simulink library "tqd"  (R2021b)
settings: Solver=VariableStepAuto  StartTime=0.0  StopTime=10.0  RelTol=1e-3
undefined symbols (not defined in the file): ATQD_AfterTqMinGain_X_Deg, ATQD_APSCreepBaseTqD_X_kph, ATQD_APSCreepBaseTqD_Y_Deg, ATQD_APSCreepBaseTqR_X_kph, ATQD_APSCreepBaseTqR_Y_Deg, ATQD_APSCreepIterm_X_kph, ATQD_APSCreepIterm_Y_kph, ATQD_APSCreepPterm_X_kph, ATQD_APSCreepPterm_Y_kph, ATQD_APSDecReq_X_kph, ATQD_APSDecReq_Y_mps2, ATQD_APSDecReqCMD_X_kph, ATQD_APSDecReqTs_X_pct, ATQD_APSDecTimeGain_X_Deg, ATQD_APSDecTimeGain_Y_s, ATQD_APSReqLowSpd_X_Deg, ATQD_AutoHoldReleaseBPS_X_Deg, ATQD_AWDLoadTrqnsGain_X_kg, ATQD_AWDLoadTrqnsGain_Y_pct, ATQD_BOSEnBPSPosn_X_kph, ATQD_BOSMap_X_rpm, ATQD_BOSMap_Y_pct, ATQD_CreepBaseTqD_X_kph, ATQD_CreepBaseTqD_Y_Deg, ATQD_CreepBaseTqR_X_kph, ATQD_CreepBaseTqR_Y_Deg, ATQD_CreepBPSDisPosn_X_Deg, ATQD_CreepBPSDisPosnR_X_Deg, ATQD_CreepBPSEnPosn_X_Deg, ATQD_CreepBPSEnPosnR_X_Deg, ATQD_CreepDeltaTq_X_kph, ATQD_CreepIterm_X_kph, ATQD_CreepIterm_Y_kph, ATQD_CreepItermMaxLimit_X_pct, ATQD_CreepPreloadTime_X_kph, ATQD_CreepPreloadTq_X_kph, ATQD_CreepPreloadTq_Y_s, ATQD_CreepProtTq_X_Deg, ATQD_CreepPterm_X_kph, ATQD_CreepPterm_Y_kph, ATQD_CreepRrTqSpRat_X_rpm, ATQD_CreepRrTqSpRat_Y_Nm, ATQD_CreepTargetSpdD_X_pct, ATQD_CreepTargetSpdR_X_pct, ATQD_ECOTqMapD_X_rpm, ATQD_ECOTqMapD_Y_pct, ATQD_EMTqMapD_X_rpm, ATQD_EMTqMapD_Y_pct, ATQD_EOPDTqMapDCon_X_rpm, ATQD_EOPDTqMapDCon_Y_Deg, ATQD_EscapeModePedTq_X_pct, ATQD_EscapeModePedTq_Y_rpm, ATQD_EscapeModePedTqFr_X_pct, ATQD_EscapeModePedTqFr_Y_rpm, ATQD_EstInitVehWeight_X_c, ATQD_FAfterTqCMDGain_X_rpm, ATQD_FAfterTqCMDGain_Y_pct, ATQD_FrLossMAPLowV_X_rpm, ATQD_FrLossMAPLowV_Y_Nm, ATQD_FrMotActReduce_X_rpm ... (+772)
libraries: simulink x211, hcu_lib x179, tqr x3
(part 26 of 28)

== stateflow chart tqd/TQD/TorqueDemand/Signal_convert/Chart ==
  state Creep_function_switch
    (default) -> (junction 12) : { VTQD_SaveCreepSW_flg =FALSE;}
    Creep_function_switch -> (junction 12)
    (junction 12) -> (junction 16) [order 1] : [VPMM_SysPowerMode_enum != ENUM_PWRSTASW_STANDBY ]
    (junction 12) -> (junction 19) [order 2] : {VTQD_CreepON_flg = TRUE;
        |  VTQD_SaveCreepSW_flg = VTQD_CreepON_flg;}
    (junction 16) -> (junction 23)
    (junction 23) -> (junction 25) [order 1] : [KTQD_CreepSW_flg_ovrdflg != TRUE]
    (junction 23) -> (junction 28) [order 2] : {VTQD_CreepON_flg = KTQD_CreepSW_flg_ovrdval;}
    (junction 25) -> (junction 30)
    (junction 30) -> (junction 32) [order 1] : [VINP_RegenMode_enum != ENUM_REGENLEVEL_OPD]
    (junction 30) -> (junction 34) [order 2] : {VTQD_CreepON_flg = FALSE;}
    (junction 32) -> (junction 37)
    (junction 37) -> (junction 39) [order 1] : [VTQD_OPDOn2Off_flg != TRUE]
    (junction 37) -> (junction 42) [order 2] : {VTQD_CreepON_flg = VTQD_SaveCreepSW_flg;}
    (junction 39) -> (junction 45)
    (junction 45) -> (junction 47) [order 1] : [VINP_IVICreepSWReq_flg == TRUE]
    (junction 45) -> (junction 49) [order 2] : {VTQD_CreepON_flg = VTQD_LastCreepON_flg;}
    (junction 47) -> (junction 51)
    (junction 51) -> (junction 53) [order 1] : [VTQD_LastCreepON_flg != FALSE]
    (junction 51) -> (junction 55) [order 2] : {VTQD_CreepON_flg = TRUE;
        |  VTQD_SaveCreepSW_flg = VTQD_CreepON_flg;}
    (junction 53) -> (junction 57) : {VTQD_CreepON_flg = FALSE;
        |  VTQD_SaveCreepSW_flg = VTQD_CreepON_flg;}
  (default) -> Creep_function_switch
  data: VPMM_SysPowerMode_enum input; KTQD_CreepSW_flg_ovrdflg input; KTQD_CreepSW_flg_ovrdval input; VTQD_OPDOn2Off_flg input; VINP_RegenMode_enum input; VTQD_LastCreepON_flg input; VINP_IVICreepSWReq_flg input; ENUM_PWRSTASW_STANDBY parameter; TRUE parameter; VTQD_CreepON_flg output boolean; ENUM_REGENLEVEL_OPD parameter; FALSE parameter; VTQD_SaveCreepSW_flg local boolean

== stateflow chart tqd/TQD/TorqueDemand/ShiftModule/Determine_Actual_Gear_Position ==
  state Initialize [commented out]
    en:
    VTQD_GearActualPosn_enum = ENUM_GEARACTUALPOSN_INVALID;
    VTQD_ShiftInitialComplete_flg = FALSE;
    (default) -> (junction 489) [commented out] : {
        | VTQD_InitializeTime_s = 0;
        | }
    Initialize -> (junction 489) [commented out]
    (junction 489) -> (junction 490) [commented out] : [VTQD_InitializeTime_s > KTQD_ShiftInitialTime_s]
    (junction 489) -> (junction 531) [commented out] : {
        | VTQD_InitializeTime_s = VTQD_InitializeTime_s + task_time_s;
        | }
    (junction 490) -> (junction 533) [commented out] : {
        | VTQD_ShiftInitialComplete_flg = TRUE;
        | }
    (junction 533) -> (junction 531) [commented out]
  state PBW_Judgement [commented out]
    en:
    VTQD_PBWReleased_flg = FALSE;
    VTQD_PBWLocked_flg = FALSE;
    VTQD_PBWUnlockTO_flg = FALSE;
    VTQD_PBWLockTO_flg = FALSE;
    state Initialize [commented out]
      en:
      VTQD_PBWUnlockTO_flg = FALSE;
      VTQD_PBWReleased_flg = FALSE;
      VTQD_PBWLocked_flg = FALSE;
    state PBWUnlock [commented out]
      en:
      VTQD_ParkRequest_flg = FALSE;
      (default) -> (junction 798) [commented out] : {
          | VTQD_PBWWaitTime_s = 0;
          | }
      PBWUnlock -> (junction 798) [commented out]
      (junction 798) -> (junction 799) [commented out] : [VINP_PBWMotorPos_enum == ENUM_PBWPOSITION_UNPARKED]
      (junction 798) -> (junction 800) [commented out] : {
          | VTQD_PBWWaitTime_s += task_time_s;
          | }
      (junction 799) -> (junction 804) [commented out] : {
          | VTQD_PBWReleased_flg = TRUE;
          | }
      (junction 800) -> (junction 801) [commented out] : [VTQD_PBWWaitTime_s >= KTQD_PBWTimeout_s]
      (junction 800) -> (junction 802) [commented out]
      (junction 801) -> (junction 803) [commented out] : {
          | VTQD_PBWUnlockTO_flg = TRUE;
          | }
      (junction 803) -> (junction 802) [commented out]
      (junction 804) -> (junction 803) [commented out]
    state PBWLock [commented out]
      en:
      VTQD_ParkRequest_flg = TRUE;
      (default) -> (junction 817) [commented out] : {
          | VTQD_PBWWaitTime_s = 0;
          | }
      (junction 817) -> (junction 816) [commented out] : [VINP_PBWMotorPos_enum == ENUM_PBWPOSITION_PARKED]
      PBWLock -> (junction 817) [commented out]
      (junction 816) -> (junction 822) [commented out] : {
          | VTQD_PBWLocked_flg = TRUE;
          | }
      (junction 817) -> (junction 818) [commented out] : {
          | VTQD_PBWWaitTime_s += task_time_s;
          | }
      (junction 818) -> (junction 819) [commented out] : [VTQD_PBWWaitTime_s >= KTQD_PBWTimeout_s]
      (junction 818) -> (junction 820) [commented out]
      (junction 819) -> (junction 821) [commented out] : {
          | VTQD_PBWLockTO_flg = TRUE;
          | }
      (junction 821) -> (junction 820) [commented out]
      (junction 822) -> (junction 821) [commented out]
    (default) -> PBW_Judgement.Initialize [commented out]
    PBW_Judgement.Initialize -> PBWUnlock [commented out] : [VTQD_GearShiftCMD_enum != ENUM_GEARSHIFTCMD_P]
    PBW_Judgement.Initialize -> PBWLock [commented out] : [VTQD_GearShiftCMD_enum == ENUM_GEARSHIFTCMD_P]
  state N
    en:
    VTQD_GearActualPosn_enum = ENUM_GEARACTUALPOSN_N;
    VTQD_ParkRequest_flg = FALSE;
    VTQD_EnterP_flg = FALSE;
    (default) -> (junction 753) : {
        | VTQD_RelockWaitTime_s = 0;
        | }
    (junction 753) -> (junction 754) [order 1] : %[!VTQD_PBWLockTO_flg]
    N -> (junction 753) [order 1]
    (junction 753) -> (junction 755) [order 2] : {
        | VTQD_RelockWaitTime_s += task_time_s;
        | }
    (junction 754) -> (junction 757) : {
        | VTQD_EnterP_flg = TRUE;
        | }
    (junction 755) -> (junction 756) [order 1] : [VTQD_RelockWaitTime_s >= KTQD_RelockWaitTime_s]
    (junction 755) -> (junction 760) [order 2]
    (junction 756) -> (junction 758) : {
        | VTQD_EnterP_flg = TRUE;
        | }
    (junction 758) -> (junction 760)
    (junction 757) -> (junction 758)
  state P
    en:
    VTQD_GearActualPosn_enum = ENUM_GEARACTUALPOSN_P;
    VTQD_ParkRequest_flg = TRUE;
    VTQD_ExitP_flg = FALSE;
    (default) -> (junction 636) : {
        | VTQD_ReunlockWaitTime_s = 0;
        | }
    P -> (junction 636) [order 1]
    (junction 636) -> (junction 641) [order 1] : %[!VTQD_PBWUnlockTO_flg]
    (junction 636) -> (junction 645) [order 2] : {
        | VTQD_ReunlockWaitTime_s += task_time_s;
        | }
    (junction 641) -> (junction 637) : {
        | VTQD_ExitP_flg = TRUE;
        | }
    (junction 645) -> (junction 632) [order 1] : [VTQD_ReunlockWaitTime_s >= KTQD_ReunlockWaitTime_s]
    (junction 645) -> (junction 647) [order 2]
    (junction 632) -> (junction 643) : {
        | VTQD_ExitP_flg = TRUE;
        | }
    (junction 643) -> (junction 647)
    (junction 637) -> (junction 643)
  state D
    en:
    VTQD_GearActualPosn_enum = ENUM_GEARACTUALPOSN_D;
    VTQD_ParkRequest_flg = FALSE;
  state R
    en:
    VTQD_GearActualPosn_enum = ENUM_GEARACTUALPOSN_R;
    VTQD_ParkRequest_flg = FALSE;
  (default) -> P : {
      |  VTQD_PBWLockTO_flg = FALSE;
      |  VTQD_PBWUnlockTO_flg = FALSE;
      | }
  N -> (junction 731) [order 2] : [VTQD_GearShiftCMD_enum == ENUM_GEARSHIFTCMD_R && VTQD_PwrStaAllowDR_flg &&...
      |  VTQD_TMRotateDirction_enum ~= ENUM_TMROTATEDIRECTACT_FORWARD &&...
      | (VTQD_BrkSwSta_flg || VVMC_APSActive_flg || VTQD_IVIRockModeEn_flg) && !VINP_EPBCarWashMode_flg]
  P -> N [order 1] : [(VTQD_GearShiftCMD_enum == ENUM_GEARSHIFTCMD_N &&...
      | VTQD_PwrStaAllowPN_flg && (VTQD_BrkSwSta_flg || VVMC_APSActive_flg) && VTQD_ExitP_flg)&&...
      | !VTQD_ForceP_flg]
  (junction 731) -> (junction 733)
  (junction 749) -> N
  N -> P [order 3] : [(VTQD_GearShiftCMD_enum == ENUM_GEARSHIFTCMD_P && VTQD_PwrStaAllowPN_flg &&...
      |  VINP_VehSpd_kph <= KTQD_VehSpd2P_kph && VTQD_EnterP_flg) || VTQD_ForceP_flg ]
  (junction 747) -> (junction 749)
  D -> N [order 1] : [VTQD_GearShiftCMD_enum == ENUM_GEARSHIFTCMD_N ||...
      | !VTQD_PwrStaAllowDR_flg ||...
      | VINP_EPBCarWashMode_flg]
  N -> D [order 1] : [VTQD_GearShiftCMD_enum == ENUM_GEARSHIFTCMD_D && VTQD_PwrStaAllowDR_flg &&...
      |  VTQD_TMRotateDirction_enum ~= ENUM_TMROTATEDIRECTACT_REVERSE &&...
      | !VINP_EPBCarWashMode_flg]
  P -> D [order 2] : [VTQD_GearShiftCMD_enum == ENUM_GEARSHIFTCMD_D &&...
      | VTQD_PwrStaAllowDR_flg && (VTQD_BrkSwSta_flg || VVMC_APSActive_flg) && VTQD_ExitP_flg &&...
      |  !VTQD_ForceP_flg]
  D -> P [order 2] : [(VTQD_GearShiftCMD_enum == ENUM_GEARSHIFTCMD_P && VTQD_PwrStaAllowPN_flg &&...
      |  VINP_VehSpd_kph <= KTQD_VehSpd2P_kph) || VTQD_ForceP_flg]
  R -> D [order 3] : [VTQD_GearShiftCMD_enum == ENUM_GEARSHIFTCMD_D && VTQD_PwrStaAllowDR_flg &&...
      | ( VTQD_BrkSwSta_flg ||VVMC_APSActive_flg || VTQD_IVIRockModeEn_flg) &&...
      | (VINP_VehSpd_kph <= KTQD_VehSpdRev_kph || (VTQD_IVIRockModeEn_flg && ...
      |  VTQD_MaxShaftSpd_rpm <= KTQD_RockVehSpdRev_rpm))]
      | %add20250331
  D -> R [order 3] : [VTQD_GearShiftCMD_enum == ENUM_GEARSHIFTCMD_R && VTQD_PwrStaAllowDR_flg &&...
      |  (VTQD_BrkSwSta_flg || VVMC_APSActive_flg || VTQD_IVIRockModeEn_flg) &&...
      | (VINP_VehSpd_kph <= KTQD_VehSpdRev_kph || (VTQD_IVIRockModeEn_flg && ...
      |  VTQD_MaxShaftSpd_rpm <= KTQD_RockVehSpdRev_rpm))]
      | %add20250331
  P -> R [order 3] : [VTQD_GearShiftCMD_enum == ENUM_GEARSHIFTCMD_R &&...
      | VTQD_PwrStaAllowDR_flg && (VTQD_BrkSwSta_flg || VVMC_APSActive_flg) && VTQD_ExitP_flg && !VTQD_ForceP_flg]
  R -> (junction 747) [order 1] : [VTQD_GearShiftCMD_enum == ENUM_GEARSHIFTCMD_N ||...
      | !VTQD_PwrStaAllowDR_flg ||...
      | VINP_EPBCarWashMode_flg]
  (junction 733) -> R
  R -> P [order 2] : [(VTQD_GearShiftCMD_enum == ENUM_GEARSHIFTCMD_P && VTQD_PwrStaAllowPN_flg &&...
      |  VINP_VehSpd_kph <= KTQD_VehSpd2P_kph) || VTQD_ForceP_flg]
  data: task_time_s input; VTQD_BrkSwSta_flg input; VTQD_GearShiftCMD_enum input; VINP_VehSpd_kph input; VINP_PBWMotorPos_enum input; VTQD_PwrStaAllowDR_flg input; VTQD_PwrStaAllowPN_flg input; VTQD_TMRotateDirction_enum input; VTQD_GearActualPosn_enum output uint8; ENUM_GEARACTUALPOSN_N parameter; ENUM_GEARACTUALPOSN_D parameter; ENUM_GEARACTUALPOSN_R parameter; ENUM_GEARACTUALPOSN_P parameter; KTQD_VehSpd2P_kph input; VTQD_InitializeTime_s local single; ENUM_GEARACTUALPOSN_INVALID parameter; FALSE parameter; TRUE parameter; VTQD_ShiftInitialComplete_flg local boolean; ENUM_GEARSHIFTCMD_D parameter; ENUM_GEARSHIFTCMD_P parameter; ENUM_GEARSHIFTCMD_R parameter; ENUM_GEARSHIFTCMD_N parameter; KTQD_VehSpdRev_kph input; KTQD_ShiftInitialTime_s input; ENUM_PBWPOSITION_PARKED parameter; ENUM_PBWPOSITION_UNPARKED parameter; VTQD_PBWLockTO_flg output boolean; VTQD_PBWUnlockTO_flg output boolean; KTQD_PBWTimeout_s input; KTQD_RelockWaitTime_s input; KTQD_ReunlockWaitTime_s input; VTQD_ParkRequest_flg output boolean; VTQD_EnterP_flg local boolean; VTQD_ExitP_flg local boolean; VTQD_PBWLocked_flg local boolean; VTQD_PBWReleased_flg local boolean; VTQD_PBWWaitTime_s local single; VTQD_RelockWaitTime_s local single; VTQD_ReunlockWaitTime_s local single; ENUM_TMROTATEDIRECTACT_FORWARD parameter; ENUM_TMROTATEDIRECTACT_REVERSE parameter; VINP_EPBCarWashMode_flg input; VVMC_APSActive_flg input; VTQD_ForceP_flg input; VTQD_IVIRockModeEn_flg input; VTQD_MaxShaftSpd_rpm input; KTQD_RockVehSpdRev_rpm parameter

== stateflow chart tqd/TQD/TorqueDemand/Signal_convert/SWC2_Subsystem/Speed Control Mode ==
  state OFF
    en:
    VTQD_SpdCtrlMode_enum = ENUM_SPDCTRLMODE_OFF;
    VTQD_SpdCtrlSta_flg = FALSE;
  state ACC
    en:
    VTQD_SpdCtrlMode_enum = ENUM_SPDCTRLMODE_ACC;
    VTQD_SpdCtrlSta_flg = TRUE;
  state MSA
    en:
    VTQD_SpdCtrlMode_enum = ENUM_SPDCTRLMODE_MSA;
    VTQD_SpdCtrlSta_flg = TRUE;
  (default) -> OFF
  (junction 117) -> OFF
  (junction 26) -> (junction 117) [order 1] : [
      |  VPMM_PowerSta_enum != ENUM_POWERSTA_READY || ...
      |  VTQD_ShiftGearPosn_enum == ENUM_GEARPOSNTOCAN_P
      | ]
  ACC -> OFF [order 1] : [
      | VPMM_PowerSta_enum != ENUM_POWERSTA_READY || ...
      | VTQD_ShiftGearPosn_enum != ENUM_GEARPOSNTOCAN_D
      | ]
  OFF -> ACC : [
      | VPMM_PowerSta_enum == ENUM_POWERSTA_READY && ...
      | VTQD_ShiftGearPosn_enum == ENUM_GEARPOSNTOCAN_D
      | ]
  (junction 26) -> ACC [order 2]
  (junction 19) -> (junction 26)
  ACC -> MSA [order 2] : [VTQD_LScrollPressLong_flg && ...
      | VVMC_MSACtrlSta_enum != ENUM_ADASMSASTA_ACTIVE]
      | %add20241210
  MSA -> (junction 19) : [
      |  VPMM_PowerSta_enum != ENUM_POWERSTA_READY || ...
      |  VTQD_ShiftGearPosn_enum == ENUM_GEARPOSNTOCAN_P ||...
      |  VTQD_SWC2LADASSta_flg
      |  ]
      | %add20241210
  data: VPMM_PowerSta_enum input; VTQD_LScrollPressLong_flg input; ENUM_SPDCTRLMODE_OFF parameter; ENUM_SPDCTRLMODE_ACC parameter; ENUM_SPDCTRLMODE_MSA parameter; FALSE parameter; ENUM_POWERSTA_READY parameter; VTQD_SpdCtrlMode_enum output uint8; VTQD_SpdCtrlSta_flg output boolean; TRUE parameter; VTQD_ShiftGearPosn_enum input; ENUM_GEARPOSNTOCAN_D parameter; ENUM_GEARPOSNTOCAN_P parameter; VTQD_SWC2LADASSta_flg input; VVMC_MSACtrlSta_enum input; ENUM_ADASMSASTA_ACTIVE parameter

== stateflow chart tqd/TQD/TorqueDemand/Signal_convert/SWC_Subsystem/Speed Setting Mode/CC Speed Setting ON/Specific_STATE_ChangeToSTANDBY ==
  state FLG_ON
    en:
    VTQD_CCChangeToSTANDBY_flg = TRUE;
  state Initialize
    en:
    VTQD_CCChangeToSTANDBY_flg = FALSE;
  state STAY
  (default) -> Initialize
  Initialize -> STAY : [VVMC_CCCtrlSta_enum == ENUM_ADASCCSTA_ACTIVE]
  STAY -> FLG_ON [order 1] : [VVMC_CCCtrlSta_enum == ENUM_ADASCCSTA_STANDBY]
  STAY -> Initialize [order 2] : [VVMC_CCCtrlSta_enum != ENUM_ADASCCSTA_ACTIVE &&...
      | VVMC_CCCtrlSta_enum != ENUM_ADASCCSTA_STANDBY ]
  (junction 11) -> Initialize
  FLG_ON -> (junction 9)
  (junction 9) -> (junction 11) : [VVMC_CCCtrlSta_enum != ENUM_ADASCCSTA_STANDBY]
  data: VVMC_CCCtrlSta_enum input; FALSE parameter; TRUE parameter; VTQD_CCChangeToSTANDBY_flg output boolean; ENUM_ADASCCSTA_ACTIVE parameter; ENUM_ADASCCSTA_STANDBY parameter

== stateflow chart tqd/TQD/TorqueDemand/Signal_convert/SWC2_Subsystem/Speed Setting Mode/ACC Speed Setting ON/ACCSetSpd_2506 ==
  state MeterSpd
    state OFF_Error_Disable
      en:
      VTQD_ACCSetSpd_raw32 =  min(VTQD_ACCActiveMetSpdHi_raw32, VTQD_SpdLim4SetSpd_raw32);
      VTQD_ACCSetSpd_raw32 = max(VTQD_ACCActiveMetSpdLo_raw32, VTQD_ACCSetSpd_raw32);
      VTQD_ACCSavedSetSpd_raw32 = VTQD_ACCSetSpd_raw32;
      du:
      VTQD_ACCSetSpd_raw32 =  min(VTQD_ACCActiveMetSpdHi_raw32, VTQD_SpdLim4SetSpd_raw32);
      VTQD_ACCSetSpd_raw32 = max(VTQD_ACCActiveMetSpdLo_raw32, VTQD_ACCSetSpd_raw32);
      VTQD_ACCSavedSetSpd_raw32 = VTQD_ACCSetSpd_raw32;
    state Terminal
      %Do Nothing
    state Standby
      en:
      VTQD_ACCSetSpd_raw32 =  min(VTQD_ACCActiveMetSpdHi_raw32, VTQD_SpdLim4SetSpd_raw32);
      VTQD_ACCSetSpd_raw32 = max(VTQD_ACCActiveMetSpdLo_raw32, VTQD_ACCSetSpd_raw32);
      VTQD_ACCSavedSetSpd_raw32 = VTQD_ACCSetSpd_raw32;
      du:
      VTQD_ACCSetSpd_raw32 =  min(VTQD_ACCActiveMetSpdHi_raw32, VTQD_SpdLim4SetSpd_raw32);
      VTQD_ACCSetSpd_raw32 = max(VTQD_ACCActiveMetSpdLo_raw32, VTQD_ACCSetSpd_raw32);
      VTQD_ACCSavedSetSpd_raw32 = VTQD_ACCSetSpd_raw32;
    state Active_Override_ShutOff
      (default) -> (junction 749) : {VTQD_HoldResDet_flg = FALSE;
          |  VTQD_ACCSavedSetSpd_raw32 = VTQD_LastSetSpd_kph;
          |  VTQD_ACCSetSpd_raw32 = VTQD_ACCSavedSetSpd_raw32}
      MeterSpd.Active_Override_ShutOff -> (junction 830) [order 1]
      (junction 830) -> (junction 834) [order 1] : [VTQD_DistanceUnit_flg == VINP_Distanceunit_flg || VTQD_ACCSavedSetSpd_raw32 <= ONE_FLOAT]
      (junction 834) -> (junction 749) : {VTQD_ACCSetSpd_raw32 = min(VTQD_ACCActiveMetSpdHi_raw32, VTQD_ACCSavedSetSpd_raw32);
          |  VTQD_ACCSavedSetSpd_raw32 = VTQD_ACCSetSpd_raw32;}
      (junction 749) -> (junction 1142) [order 1] : [VINP_ADASACCSta_enum == ENUM_ADASACCSTA_ACTIVE]
      (junction 1142) -> (junction 1148) [order 1] : [(VTQD_SWC2ScrollUpSta_flg ||...
          |   VTQD_SWC2ScrollDownSta_flg ||...
          |   VTQD_SWC2ScrollUpSta_enum == ENUM_SWCBOTTONPRESS_SHORTPRESS ||...
          |   VTQD_SWC2ScrollDownSta_enum == ENUM_SWCBOTTONPRESS_SHORTPRESS) &&...
          |  VTQD_HoldResDet_flg]
          | %add20250114
      (junction 830) -> (junction 832) [order 2]
      (junction 837) -> (junction 834)
      (junction 749) -> (junction 798) [order 2]
      (junction 1142) -> (junction 1144) [order 2] : {VTQD_HoldResDet_flg = FALSE}
          | %add20250114
      (junction 1148) -> (junction 1146) : {VTQD_HoldResDet_flg = TRUE}
          | %add20250114
      (junction 832) -> (junction 819) [order 1] : [VINP_Distanceunit_flg]
      (junction 832) -> (junction 833) [order 2] : {VTQD_ACCSavedSetSpd_raw32 = (VTQD_ACCSavedSetSpd_raw32 * MPH2KPH)}
      (junction 819) -> (junction 827) : {VTQD_ACCSavedSetSpd_raw32 = (VTQD_ACCSavedSetSpd_raw32 * KPH2MPH)}
      (junction 1144) -> (junction 1146)
      (junction 1146) -> (junction 751)
      (junction 751) -> (junction 757) [order 1] : [VTQD_Set2MeterSpd_flg ||...
          |  VTQD_SetRoadSpdLim_flg]
      (junction 757) -> (junction 1115) [order 1] : [VTQD_Set2MeterSpd_flg]
      (junction 751) -> (junction 762) [order 2]
      (junction 757) -> (junction 759) [order 2] : {VTQD_ACCSetSpd_raw32 =  min(VTQD_ACCActiveMetSpdHi_raw32, VTQD_SpdLim4SetSpd_raw32);
          |  VTQD_ACCSetSpd_raw32 = max(VTQD_ACCActiveMetSpdLo_raw32, VTQD_ACCSetSpd_raw32);
          |  VTQD_ACCSavedSetSpd_raw32 = VTQD_ACCSetSpd_raw32;
          |  VTQD_DistanceUnit_flg = VINP_Distanceunit_flg;}
      (junction 1115) -> (junction 1114) : {VTQD_ACCSetSpd_raw32 =  min(VTQD_ACCActiveMetSpdHi_raw32, VVMC_MeterIndSpeed_raw32);
          |  VTQD_ACCSetSpd_raw32 = max(VTQD_ACCActiveMetSpdLo_raw32, VTQD_ACCSetSpd_raw32);
          |  VTQD_ACCSavedSetSpd_raw32 = VTQD_ACCSetSpd_raw32;
          |  VTQD_DistanceUnit_flg = VINP_Distanceunit_flg;}
      (junction 827) -> (junction 816) [order 1] : [VTQD_ACCSavedSetSpd_raw32 < KTQD_ACCActiveMetSpdLoMPH_mph]
      (junction 833) -> (junction 817) [order 1] : [VTQD_ACCSavedSetSpd_raw32 < KTQD_ACCActiveMetSpdLo_kph]
      (junction 816) -> (junction 820) : {VTQD_ACCSavedSetSpd_raw32 = KTQD_ACCActiveMetSpdLoMPH_mph}
      (junction 833) -> (junction 828) [order 2]
      (junction 817) -> (junction 815) : {VTQD_ACCSavedSetSpd_raw32 = KTQD_ACCActiveMetSpdLo_kph}
      (junction 827) -> (junction 818) [order 2]
      (junction 820) -> (junction 818)
      (junction 815) -> (junction 828)
      (junction 818) -> (junction 826)
      (junction 828) -> (junction 821)
      (junction 762) -> (junction 766) [order 1] : [(VTQD_SWC2ScrollUpSta_enum == ENUM_SWCBOTTONPRESS_SHORTPRESS ||...
          |   VTQD_SWC2ScrollDownSta_enum == ENUM_SWCBOTTONPRESS_SHORTPRESS) &&...
          |  !VVMC_LVDAACCStatusInformation_flg && !VTQD_HoldResDet_flg]
          | %add20250114
      (junction 766) -> (junction 771) [order 1] : [VTQD_SWC2ScrollUpSta_enum == ENUM_SWCBOTTONPRESS_SHORTPRESS]
      (junction 821) -> (junction 829) [order 1] : [VTQD_ACCSavedSetSpd_raw32 > KTQD_ACCActiveMetSpdHi_kph]
      (junction 826) -> (junction 822) [order 1] : [VTQD_ACCSavedSetSpd_raw32 > KTQD_ACCActiveMetSpdHiMPH_mph]
      (junction 762) -> (junction 792) [order 2]
      (junction 766) -> (junction 779) [order 2] : {VTQD_ACCSetSpd_raw32 =  min(VTQD_ACCActiveMetSpdHi_raw32, VTQD_ACCSavedSetSpd_raw32 - ONE_FLOAT);
          |  VTQD_ACCSetSpd_raw32 = max(VTQD_ACCActiveMetSpdLo_raw32, VTQD_ACCSetSpd_raw32);
          |  VTQD_ACCSavedSetSpd_raw32 = VTQD_ACCSetSpd_raw32;
          |  VTQD_DistanceUnit_flg = VINP_Distanceunit_flg;}
      (junction 771) -> (junction 774) : {VTQD_ACCSetSpd_raw32 =  min(VTQD_ACCActiveMetSpdHi_raw32, VTQD_ACCSavedSetSpd_raw32 + ONE_FLOAT);
          |  VTQD_ACCSetSpd_raw32 = max(VTQD_ACCActiveMetSpdLo_raw32, VTQD_ACCSetSpd_raw32);
          |  VTQD_ACCSavedSetSpd_raw32 = VTQD_ACCSetSpd_raw32;
          |  VTQD_DistanceUnit_flg = VINP_Distanceunit_flg;}
      (junction 821) -> (junction 823) [order 2]
      (junction 829) -> (junction 831) : {VTQD_ACCSavedSetSpd_raw32 = KTQD_ACCActiveMetSpdHi_kph}
      (junction 826) -> (junction 835) [order 2]
      (junction 822) -> (junction 824) : {VTQD_ACCSavedSetSpd_raw32 = KTQD_ACCActiveMetSpdHiMPH_mph}
      (junction 831) -> (junction 823)
      (junction 824) -> (junction 835)
      (junction 823) -> (junction 825)
      (junction 835) -> (junction 836)
      (junction 825) -> (junction 836)
      (junction 836) -> (junction 837)
      (junction 792) -> (junction 785) [order 1] : [(VTQD_SWC2ScrollUpSta_enum == ENUM_SWCBOTTONPRESS_LONGPRESS ||...
          |   VTQD_SWC2ScrollDownSta_enum == ENUM_SWCBOTTONPRESS_LONGPRESS) &&...
          |  !VVMC_LVDAACCStatusInformation_flg && !VTQD_HoldResDet_flg]
          | %add20250114
      (junction 785) -> (junction 790) [order 1] : [VTQD_SWC2ScrollUpSta_enum == ENUM_SWCBOTTONPRESS_LONGPRESS]
      (junction 792) -> (junction 1131) [order 2]
      (junction 785) -> (junction 793) [order 2] : {VTQD_ACCSetSpd_raw32 = max(VTQD_ACCActiveMetSpdLo_raw32, ceil(VTQD_ACCSavedSetSpd_raw32 / VTQD_SetSpdDeltaLong_raw32 - ONE_FLOAT) * VTQD_SetSpdDeltaLong_raw32);
          |  VTQD_ACCSetSpd_raw32 = min (VTQD_ACCActiveMetSpdHi_raw32, VTQD_ACCSetSpd_raw32);
          |  VTQD_ACCSavedSetSpd_raw32 = VTQD_ACCSetSpd_raw32;
          |  VTQD_DistanceUnit_flg = VINP_Distanceunit_flg;}
      (junction 790) -> (junction 783) : {VTQD_ACCSetSpd_raw32 = min(VTQD_ACCActiveMetSpdHi_raw32, floor(VTQD_ACCSavedSetSpd_raw32 / VTQD_SetSpdDeltaLong_raw32 + ONE_FLOAT) * VTQD_SetSpdDeltaLong_raw32);
          |  VTQD_ACCSetSpd_raw32 = max (VTQD_ACCActiveMetSpdLo_raw32, VTQD_ACCSetSpd_raw32);
          |  VTQD_ACCSavedSetSpd_raw32 = VTQD_ACCSetSpd_raw32;
          |  VTQD_DistanceUnit_flg = VINP_Distanceunit_flg;}
      (junction 1131) -> (junction 1133) [order 1] : [(VTQD_SWC2ScrollUpSta_flg ||...
          |   VTQD_SWC2ScrollDownSta_flg) &&...
          |  VVMC_LVDAACCStatusInformation_flg]
          | %add20250114
      (junction 1131) -> (junction 1137) [order 2]
      (junction 1133) -> (junction 1134) : {VTQD_HoldResDet_flg = TRUE}
          | %add20250114
      (junction 1134) -> (junction 1137)
      (junction 1137) -> (junction 1265) : {VTQD_ACCSetSpd_raw32 = VTQD_ACCSavedSetSpd_raw32;
          |  VTQD_ACCSavedSetSpd_raw32 = VTQD_ACCSetSpd_raw32;
          |  VTQD_DistanceUnit_flg = VINP_Distanceunit_flg;}
      (junction 798) -> (junction 1240) [order 1] : [VINP_ADASACCSta_enum == ENUM_ADASACCSTA_OVERRIDE]
      (junction 1240) -> (junction 1235) [order 1] : [KTQD_ACCOVRDSpdAdj_flg &&...
          | (VTQD_Set2MeterSpd_flg ||...
          |  VTQD_SetRoadSpdLim_flg)]
      (junction 1235) -> (junction 1247) [order 1] : [VTQD_Set2MeterSpd_flg]
      (junction 798) -> (junction 807) [order 2] : {VTQD_ACCSetSpd_raw32 = VTQD_ACCSavedSetSpd_raw32;
          |  VTQD_ACCSavedSetSpd_raw32 = VTQD_ACCSetSpd_raw32;
          |  VTQD_DistanceUnit_flg = VINP_Distanceunit_flg;}
      (junction 1240) -> (junction 1236) [order 2]
      (junction 1235) -> (junction 1244) [order 2] : {VTQD_ACCSetSpd_raw32 =  min(VTQD_ACCActiveMetSpdHi_raw32, VTQD_SpdLim4SetSpd_raw32);
          |  VTQD_ACCSetSpd_raw32 = max(VTQD_ACCActiveMetSpdLo_raw32, VTQD_ACCSetSpd_raw32);
          |  VTQD_ACCSavedSetSpd_raw32 = VTQD_ACCSetSpd_raw32;
          |  VTQD_DistanceUnit_flg = VINP_Distanceunit_flg;}
      (junction 1247) -> (junction 1241) : {VTQD_ACCSetSpd_raw32 =  min(VTQD_ACCActiveMetSpdHi_raw32, VVMC_MeterIndSpeed_raw32);
          |  VTQD_ACCSetSpd_raw32 = max(VTQD_ACCActiveMetSpdLo_raw32, VTQD_ACCSetSpd_raw32);
          |  VTQD_ACCSavedSetSpd_raw32 = VTQD_ACCSetSpd_raw32;
          |  VTQD_DistanceUnit_flg = VINP_Distanceunit_flg;}
      (junction 1236) -> (junction 1242) [order 1] : [(VTQD_SWC2ScrollUpSta_enum == ENUM_SWCBOTTONPRESS_SHORTPRESS ||...
          |   VTQD_SWC2ScrollDownSta_enum == ENUM_SWCBOTTONPRESS_SHORTPRESS)]
      (junction 1242) -> (junction 1238) [order 1] : [VTQD_SWC2ScrollUpSta_enum == ENUM_SWCBOTTONPRESS_SHORTPRESS]
      (junction 1236) -> (junction 1245) [order 2]
      (junction 1242) -> (junction 1248) [order 2] : {VTQD_ACCSetSpd_raw32 =  min(VTQD_ACCActiveMetSpdHi_raw32, VTQD_ACCSavedSetSpd_raw32 - ONE_FLOAT);
          |  VTQD_ACCSetSpd_raw32 = max(VTQD_ACCActiveMetSpdLo_raw32, VTQD_ACCSetSpd_raw32);
          |  VTQD_ACCSavedSetSpd_raw32 = VTQD_ACCSetSpd_raw32;
          |  VTQD_DistanceUnit_flg = VINP_Distanceunit_flg;}
      (junction 1238) -> (junction 1239) : {VTQD_ACCSetSpd_raw32 =  min(VTQD_ACCActiveMetSpdHi_raw32, VTQD_ACCSavedSetSpd_raw32 + ONE_FLOAT);
          |  VTQD_ACCSetSpd_raw32 = max(VTQD_ACCActiveMetSpdLo_raw32, VTQD_ACCSetSpd_raw32);
          |  VTQD_ACCSavedSetSpd_raw32 = VTQD_ACCSetSpd_raw32;
          |  VTQD_DistanceUnit_flg = VINP_Distanceunit_flg;}
      (junction 1245) -> (junction 1249) [order 1] : [(VTQD_SWC2ScrollUpSta_enum == ENUM_SWCBOTTONPRESS_LONGPRESS ||...
          |   VTQD_SWC2ScrollDownSta_enum == ENUM_SWCBOTTONPRESS_LONGPRESS)]
      (junction 1249) -> (junction 1243) [order 1] : [VTQD_SWC2ScrollUpSta_enum == ENUM_SWCBOTTONPRESS_LONGPRESS]
      (junction 1245) -> (junction 1234) [order 2] : {VTQD_ACCSetSpd_raw32 = VTQD_ACCSavedSetSpd_raw32;
          |  VTQD_ACCSavedSetSpd_raw32 = VTQD_ACCSetSpd_raw32;
          |  VTQD_DistanceUnit_flg = VINP_Distanceunit_flg;}
      (junction 1249) -> (junction 1246) [order 2] : {VTQD_ACCSetSpd_raw32 = max(VTQD_ACCActiveMetSpdLo_raw32, ceil(VTQD_ACCSavedSetSpd_raw32 / VTQD_SetSpdDeltaLong_raw32 - ONE_FLOAT) * VTQD_SetSpdDeltaLong_raw32);
          |  VTQD_ACCSetSpd_raw32 = min (VTQD_ACCActiveMetSpdHi_raw32, VTQD_ACCSetSpd_raw32);
          |  VTQD_ACCSavedSetSpd_raw32 = VTQD_ACCSetSpd_raw32;
          |  VTQD_DistanceUnit_flg = VINP_Distanceunit_flg;}
      (junction 1243) -> (junction 1237) : {VTQD_ACCSetSpd_raw32 = min(VTQD_ACCActiveMetSpdHi_raw32, floor(VTQD_ACCSavedSetSpd_raw32 / VTQD_SetSpdDeltaLong_raw32 + ONE_FLOAT) * VTQD_SetSpdDeltaLong_raw32);
          |  VTQD_ACCSetSpd_raw32 = max (VTQD_ACCActiveMetSpdLo_raw32, VTQD_ACCSetSpd_raw32);
          |  VTQD_ACCSavedSetSpd_raw32 = VTQD_ACCSetSpd_raw32;
          |  VTQD_DistanceUnit_flg = VINP_Distanceunit_flg;}
    (default) -> MeterSpd.OFF_Error_Disable [order 3]
    MeterSpd.Terminal -> MeterSpd.OFF_Error_Disable [order 2] : [VINP_ADASACCSta_enum ~= ENUM_ADASACCSTA_ACTIVE &&...
        |  VINP_ADASACCSta_enum ~= ENUM_ADASACCSTA_OVERRIDE &&...
        |  VINP_ADASACCSta_enum ~= ENUM_ADASACCSTA_SHUTOFF]
    MeterSpd.OFF_Error_Disable -> MeterSpd.Terminal [order 2] : [VINP_ADASACCSta_enum == ENUM_ADASACCSTA_ACTIVE ||...
        |  VINP_ADASACCSta_enum == ENUM_ADASACCSTA_OVERRIDE ||...
        |  VINP_ADASACCSta_enum == ENUM_ADASACCSTA_SHUTOFF]
    MeterSpd.Terminal -> MeterSpd.Active_Override_ShutOff [order 1] : [VINP_ADASACCSta_enum == ENUM_ADASACCSTA_ACTIVE ||...
        |  VINP_ADASACCSta_enum == ENUM_ADASACCSTA_OVERRIDE ||...
        |  VINP_ADASACCSta_enum == ENUM_ADASACCSTA_SHUTOFF]
    MeterSpd.Active_Override_ShutOff -> MeterSpd.Terminal [order 2] : [VINP_ADASACCSta_enum ~= ENUM_ADASACCSTA_ACTIVE &&...
        |  VINP_ADASACCSta_enum ~= ENUM_ADASACCSTA_OVERRIDE &&...
        |  VINP_ADASACCSta_enum ~= ENUM_ADASACCSTA_SHUTOFF]
    MeterSpd.OFF_Error_Disable -> MeterSpd.Standby [order 1] : [VINP_ADASACCSta_enum == ENUM_ADASACCSTA_STANDBY]
    MeterSpd.Standby -> MeterSpd.OFF_Error_Disable [order 2] : [VINP_ADASACCSta_enum ~= ENUM_ADASACCSTA_STANDBY]
    MeterSpd.Active_Override_ShutOff -> MeterSpd.Standby [order 1] : [VINP_ADASACCSta_enum == ENUM_ADASACCSTA_STANDBY]
    MeterSpd.Standby -> MeterSpd.Active_Override_ShutOff [order 1] : [VINP_ADASACCSta_enum == ENUM_ADASACCSTA_ACTIVE ||...
        |  VINP_ADASACCSta_enum == ENUM_ADASACCSTA_OVERRIDE ||...
        |  VINP_ADASACCSta_enum == ENUM_ADASACCSTA_SHUTOFF]
    (default) -> MeterSpd.Active_Override_ShutOff [order 2] : [VINP_ADASACCSta_enum == ENUM_ADASACCSTA_ACTIVE ||...
        |  VINP_ADASACCSta_enum == ENUM_ADASACCSTA_OVERRIDE ||...
        |  VINP_ADASACCSta_enum == ENUM_ADASACCSTA_SHUTOFF]
    (default) -> MeterSpd.Standby [order 1] : [VINP_ADASACCSta_enum == ENUM_ADASACCSTA_STANDBY]
  state RoadSpd
    state OFF_Error_Disable
      en:
      VTQD_ACCSetSpd_raw32 =  min(VTQD_ACCActiveMetSpdHi_raw32, VTQD_SpdLim4SetSpd_raw32);
      VTQD_ACCSetSpd_raw32 = max(VTQD_ACCActiveMetSpdLo_raw32, VTQD_ACCSetSpd_raw32);
      VTQD_ACCSavedSetSpd_raw32 = VTQD_ACCSetSpd_raw32;
      du:
      VTQD_ACCSetSpd_raw32 =  min(VTQD_ACCActiveMetSpdHi_raw32, VTQD_SpdLim4SetSpd_raw32);
      VTQD_ACCSetSpd_raw32 = max(VTQD_ACCActiveMetSpdLo_raw32, VTQD_ACCSetSpd_raw32);
      VTQD_ACCSavedSetSpd_raw32 = VTQD_ACCSetSpd_raw32;
    state Terminal
      %Do Nothing
    state Standby
      (default) -> (junction 987) : {VTQD_StandbyDisRoadSpd_flg = FALSE;}
      RoadSpd.Standby -> (junction 1029) [order 1]
      (junction 1029) -> (junction 1030) [order 1] : [VTQD_DistanceUnit_flg == VINP_Distanceunit_flg || VTQD_ACCSavedSetSpd_raw32 <= ONE_FLOAT]
      (junction 1030) -> (junction 987) : {VTQD_ACCSetSpd_raw32 = min(VTQD_ACCActiveMetSpdHi_raw32, VTQD_ACCSavedSetSpd_raw32);
          |  VTQD_ACCSavedSetSpd_raw32 = VTQD_ACCSetSpd_raw32;}
      (junction 987) -> (junction 1102) [order 1] : [VTQD_RoadSpdActive2Standby_flg &&...
          | (VTQD_StandbyDisRoadSpd_flg || !VTQD_ADASSLIFSpdLimDet_flg)]
      (junction 1029) -> (junction 1031) [order 2]
      (junction 1048) -> (junction 1030)
      (junction 987) -> (junction 1104) [order 2]
      (junction 1102) -> (junction 999)
      (junction 1031) -> (junction 1032) [order 1] : [VINP_Distanceunit_flg]
      (junction 1031) -> (junction 1034) [order 2] : {VTQD_ACCSavedSetSpd_raw32 = (VTQD_ACCSavedSetSpd_raw32 * MPH2KPH)}
      (junction 1032) -> (junction 1028) : {VTQD_ACCSavedSetSpd_raw32 = (VTQD_ACCSavedSetSpd_raw32 * KPH2MPH)}
      (junction 1104) -> (junction 999) [order 1] : [VTQD_SWC2ScrollUpSta_enum ~= ENUM_SWCBOTTONPRESS_NOPRESS ||...
          |  VTQD_SWC2ScrollDownSta_enum ~= ENUM_SWCBOTTONPRESS_NOPRESS ||...
          |  VTQD_StandbyDisRoadSpd_flg]
      (junction 999) -> (junction 1000) [order 1] : [VTQD_SWC2ScrollUpSta_enum == ENUM_SWCBOTTONPRESS_SHORTPRESS ||...
          |  VTQD_SWC2ScrollDownSta_enum == ENUM_SWCBOTTONPRESS_SHORTPRESS]
      (junction 1000) -> (junction 1001) [order 1] : [VTQD_SWC2ScrollUpSta_enum == ENUM_SWCBOTTONPRESS_SHORTPRESS]
      (junction 1104) -> (junction 991) [order 2] : {VTQD_ACCSetSpd_raw32 =  min(VTQD_ACCActiveMetSpdHi_raw32, VTQD_SpdLim4SetSpd_raw32);
          |  VTQD_ACCSetSpd_raw32 = max(VTQD_ACCActiveMetSpdLo_raw32, VTQD_ACCSetSpd_raw32);
          |  VTQD_ACCSavedSetSpd_raw32 = VTQD_ACCSetSpd_raw32;
          |  VTQD_DistanceUnit_flg = VINP_Distanceunit_flg;
          |  VTQD_RoadSpdActive2Standby_flg = FALSE;}
      (junction 999) -> (junction 1007) [order 2]
      (junction 1000) -> (junction 1005) [order 2] : {VTQD_ACCSetSpd_raw32 =  min(VTQD_ACCActiveMetSpdHi_raw32, VTQD_ACCSavedSetSpd_raw32 - ONE_FLOAT);
          |  VTQD_ACCSetSpd_raw32 = max(VTQD_ACCActiveMetSpdLo_raw32, VTQD_ACCSetSpd_raw32);
          |  VTQD_ACCSavedSetSpd_raw32 = VTQD_ACCSetSpd_raw32;
          |  VTQD_DistanceUnit_flg = VINP_Distanceunit_flg;
          |  VTQD_StandbyDisRoadSpd_flg = TRUE;}
      (junction 1001) -> (junction 1006) : {VTQD_ACCSetSpd_raw32 =  min(VTQD_ACCActiveMetSpdHi_raw32, VTQD_ACCSavedSetSpd_raw32 + ONE_FLOAT);
          |  VTQD_ACCSetSpd_raw32 = max(VTQD_ACCActiveMetSpdLo_raw32, VTQD_ACCSetSpd_raw32);
          |  VTQD_ACCSavedSetSpd_raw32 = VTQD_ACCSetSpd_raw32;
          |  VTQD_DistanceUnit_flg = VINP_Distanceunit_flg;
          |  VTQD_StandbyDisRoadSpd_flg = TRUE;}
      (junction 1028) -> (junction 1033) [order 1] : [VTQD_ACCSavedSetSpd_raw32 < KTQD_ACCActiveMetSpdLoMPH_mph]
      (junction 1034) -> (junction 1035) [order 1] : [VTQD_ACCSavedSetSpd_raw32 < KTQD_ACCActiveMetSpdLo_kph]
      (junction 1033) -> (junction 1043) : {VTQD_ACCSavedSetSpd_raw32 = KTQD_ACCActiveMetSpdLoMPH_mph}
      (junction 1034) -> (junction 1038) [order 2]
      (junction 1035) -> (junction 1039) : {VTQD_ACCSavedSetSpd_raw32 = KTQD_ACCActiveMetSpdLo_kph}
      (junction 1028) -> (junction 1045) [order 2]
      (junction 1043) -> (junction 1045)
      (junction 1039) -> (junction 1038)
      (junction 1045) -> (junction 1042)
      (junction 1038) -> (junction 1040)
      (junction 1040) -> (junction 1041) [order 1] : [VTQD_ACCSavedSetSpd_raw32 > KTQD_ACCActiveMetSpdHi_kph]
      (junction 1042) -> (junction 1044) [order 1] : [VTQD_ACCSavedSetSpd_raw32 > KTQD_ACCActiveMetSpdHiMPH_mph]
      (junction 1040) -> (junction 1053) [order 2]
      (junction 1041) -> (junction 1049) : {VTQD_ACCSavedSetSpd_raw32 = KTQD_ACCActiveMetSpdHi_kph}
      (junction 1042) -> (junction 1054) [order 2]
      (junction 1044) -> (junction 1047) : {VTQD_ACCSavedSetSpd_raw32 = KTQD_ACCActiveMetSpdHiMPH_mph}
      (junction 1007) -> (junction 1011) [order 1] : [VTQD_SWC2ScrollUpSta_enum == ENUM_SWCBOTTONPRESS_LONGPRESS ||...
          |  VTQD_SWC2ScrollDownSta_enum == ENUM_SWCBOTTONPRESS_LONGPRESS]
      (junction 1011) -> (junction 1009) [order 1] : [VTQD_SWC2ScrollUpSta_enum == ENUM_SWCBOTTONPRESS_LONGPRESS]
      (junction 1007) -> (junction 1012) [order 2]
      (junction 1011) -> (junction 1010) [order 2] : {VTQD_ACCSetSpd_raw32 = max(VTQD_ACCActiveMetSpdLo_raw32, ceil(VTQD_ACCSavedSetSpd_raw32 / VTQD_SetSpdDeltaLong_raw32 - ONE_FLOAT) * VTQD_SetSpdDeltaLong_raw32);
          |  VTQD_ACCSetSpd_raw32 = min (VTQD_ACCActiveMetSpdHi_raw32, VTQD_ACCSetSpd_raw32);
          |  VTQD_ACCSavedSetSpd_raw32 = VTQD_ACCSetSpd_raw32;
          |  VTQD_DistanceUnit_flg = VINP_Distanceunit_flg;
          |  VTQD_StandbyDisRoadSpd_flg = TRUE;}
      (junction 1009) -> (junction 1008) : {VTQD_ACCSetSpd_raw32 = min(VTQD_ACCActiveMetSpdHi_raw32, floor(VTQD_ACCSavedSetSpd_raw32 / VTQD_SetSpdDeltaLong_raw32 + ONE_FLOAT) * VTQD_SetSpdDeltaLong_raw32);
          |  VTQD_ACCSetSpd_raw32 = max (VTQD_ACCActiveMetSpdLo_raw32, VTQD_ACCSetSpd_raw32);
          |  VTQD_ACCSavedSetSpd_raw32 = VTQD_ACCSetSpd_raw32;
          |  VTQD_DistanceUnit_flg = VINP_Distanceunit_flg;
          |  VTQD_StandbyDisRoadSpd_flg = TRUE;}
      (junction 1049) -> (junction 1053)
      (junction 1047) -> (junction 1054)
      (junction 1053) -> (junction 1046)
      (junction 1054) -> (junction 1050)
      (junction 1046) -> (junction 1050)
      (junction 1050) -> (junction 1048)
      (junction 1012) -> (junction 1023) [order 1] : [VTQD_LScrollPressShort_flg &&...
          |  VTQD_ADASSLIFSpdLimDet_flg]
      (junction 1023) -> (junction 1026) : {VTQD_ACCSetSpd_raw32 =  min(VTQD_ACCActiveMetSpdHi_raw32, VTQD_SpdLim4SetSpd_raw32);
          |  VTQD_ACCSetSpd_raw32 = max(VTQD_ACCActiveMetSpdLo_raw32, VTQD_ACCSetSpd_raw32);
          |  VTQD_ACCSavedSetSpd_raw32 = VTQD_ACCSetSpd_raw32;
          |  VTQD_DistanceUnit_flg = VINP_Distanceunit_flg;
          |  VTQD_StandbyDisRoadSpd_flg = FALSE;
          |  VTQD_RoadSpdActive2Standby_flg = FALSE;}
      (junction 1012) -> (junction 1022) [order 2] : {VTQD_ACCSetSpd_raw32 =  VTQD_ACCSavedSetSpd_raw32;
          |  VTQD_ACCSavedSetSpd_raw32 = VTQD_ACCSetSpd_raw32;
          |  VTQD_DistanceUnit_flg = VINP_Distanceunit_flg;}
    state Active_Override_ShutOff
      (default) -> (junction 883) : {VTQD_HoldResDet_flg = FALSE;
          |  VTQD_ACCSavedSetSpd_raw32 = VTQD_LastSetSpd_kph;
          |  VTQD_ACCSetSpd_raw32 = VTQD_ACCSavedSetSpd_raw32}
      RoadSpd.Active_Override_ShutOff -> (junction 881) [order 1]
      (junction 881) -> (junction 882) [order 1] : [VTQD_DistanceUnit_flg == VINP_Distanceunit_flg || VTQD_ACCSavedSetSpd_raw32 <= ONE_FLOAT]
      (junction 882) -> (junction 883) : {VTQD_ACCSetSpd_raw32 = min(VTQD_ACCActiveMetSpdHi_raw32, VTQD_ACCSavedSetSpd_raw32);
          |  VTQD_ACCSavedSetSpd_raw32 = VTQD_ACCSetSpd_raw32;}
      (junction 883) -> (junction 1190) [order 1] : [VINP_ADASACCSta_enum == ENUM_ADASACCSTA_ACTIVE]
      (junction 1190) -> (junction 1197) [order 1] : [(VTQD_SWC2ScrollUpSta_flg ||...
          |   VTQD_SWC2ScrollDownSta_flg ||...
          |   VTQD_SWC2ScrollUpSta_enum == ENUM_SWCBOTTONPRESS_SHORTPRESS ||...
          |   VTQD_SWC2ScrollDownSta_enum == ENUM_SWCBOTTONPRESS_SHORTPRESS) &&...
          |  VTQD_HoldResDet_flg]
          | %add20250114
      (junction 881) -> (junction 886) [order 2]
      (junction 915) -> (junction 882)
      (junction 883) -> (junction 919) [order 2]
      (junction 1190) -> (junction 1193) [order 2] : {VTQD_HoldResDet_flg = FALSE}
          | %add20250114
      (junction 1197) -> (junction 1195) : {VTQD_HoldResDet_flg = TRUE}
          | %add20250114
      (junction 886) -> (junction 887) [order 1] : [VINP_Distanceunit_flg]
      (junction 886) -> (junction 893) [order 2] : {VTQD_ACCSavedSetSpd_raw32 = (VTQD_ACCSavedSetSpd_raw32 * MPH2KPH)}
      (junction 887) -> (junction 895) : {VTQD_ACCSavedSetSpd_raw32 = (VTQD_ACCSavedSetSpd_raw32 * KPH2MPH)}
      (junction 1193) -> (junction 1195)
      (junction 1195) -> (junction 884)
      (junction 884) -> (junction 885) [order 1] : [VTQD_Set2MeterSpd_flg ||...
          |  VTQD_SetRoadSpdLim_flg]
      (junction 885) -> (junction 1124) [order 1] : [VTQD_Set2MeterSpd_flg]
      (junction 884) -> (junction 889) [order 2]
      (junction 885) -> (junction 888) [order 2] : {VTQD_ACCSetSpd_raw32 =  min(VTQD_ACCActiveMetSpdHi_raw32, VTQD_SpdLim4SetSpd_raw32);
          |  VTQD_ACCSetSpd_raw32 = max(VTQD_ACCActiveMetSpdLo_raw32, VTQD_ACCSetSpd_raw32);
          |  VTQD_ACCSavedSetSpd_raw32 = VTQD_ACCSetSpd_raw32;
          |  VTQD_DistanceUnit_flg = VINP_Distanceunit_flg;}
      (junction 1124) -> (junction 1123) : {VTQD_ACCSetSpd_raw32 =  min(VTQD_ACCActiveMetSpdHi_raw32, VVMC_MeterIndSpeed_raw32);
          |  VTQD_ACCSetSpd_raw32 = max(VTQD_ACCActiveMetSpdLo_raw32, VTQD_ACCSetSpd_raw32);
          |  VTQD_ACCSavedSetSpd_raw32 = VTQD_ACCSetSpd_raw32;
          |  VTQD_DistanceUnit_flg = VINP_Distanceunit_flg;}
      (junction 895) -> (junction 892) [order 1] : [VTQD_ACCSavedSetSpd_raw32 < KTQD_ACCActiveMetSpdLoMPH_mph]
      (junction 893) -> (junction 894) [order 1] : [VTQD_ACCSavedSetSpd_raw32 < KTQD_ACCActiveMetSpdLo_kph]
      (junction 892) -> (junction 897) : {VTQD_ACCSavedSetSpd_raw32 = KTQD_ACCActiveMetSpdLoMPH_mph}
      (junction 893) -> (junction 898) [order 2]
      (junction 894) -> (junction 899) : {VTQD_ACCSavedSetSpd_raw32 = KTQD_ACCActiveMetSpdLo_kph}
      (junction 895) -> (junction 896) [order 2]
      (junction 897) -> (junction 896)
      (junction 899) -> (junction 898)
      (junction 896) -> (junction 902)
      (junction 898) -> (junction 900)
      (junction 889) -> (junction 890) [order 1] : [(VTQD_SWC2ScrollUpSta_enum == ENUM_SWCBOTTONPRESS_SHORTPRESS ||...
          |   VTQD_SWC2ScrollDownSta_enum == ENUM_SWCBOTTONPRESS_SHORTPRESS) &&...
          |  !VVMC_LVDAACCStatusInformation_flg && !VTQD_HoldResDet_flg]
          | %add20250114
      (junction 890) -> (junction 891) [order 1] : [VTQD_SWC2ScrollUpSta_enum == ENUM_SWCBOTTONPRESS_SHORTPRESS]
      (junction 900) -> (junction 901) [order 1] : [VTQD_ACCSavedSetSpd_raw32 > KTQD_ACCActiveMetSpdHi_kph]
      (junction 902) -> (junction 903) [order 1] : [VTQD_ACCSavedSetSpd_raw32 > KTQD_ACCActiveMetSpdHiMPH_mph]
      (junction 889) -> (junction 906) [order 2]
      (junction 890) -> (junction 904) [order 2] : {VTQD_ACCSetSpd_raw32 =  min(VTQD_ACCActiveMetSpdHi_raw32, VTQD_ACCSavedSetSpd_raw32 - ONE_FLOAT);
          |  VTQD_ACCSetSpd_raw32 = max(VTQD_ACCActiveMetSpdLo_raw32, VTQD_ACCSetSpd_raw32);
          |  VTQD_ACCSavedSetSpd_raw32 = VTQD_ACCSetSpd_raw32;
          |  VTQD_DistanceUnit_flg = VINP_Distanceunit_flg;}
      (junction 891) -> (junction 905) : {VTQD_ACCSetSpd_raw32 =  min(VTQD_ACCActiveMetSpdHi_raw32, VTQD_ACCSavedSetSpd_raw32 + ONE_FLOAT);
          |  VTQD_ACCSetSpd_raw32 = max(VTQD_ACCActiveMetSpdLo_raw32, VTQD_ACCSetSpd_raw32);
          |  VTQD_ACCSavedSetSpd_raw32 = VTQD_ACCSetSpd_raw32;
          |  VTQD_DistanceUnit_flg = VINP_Distanceunit_flg;}
      (junction 900) -> (junction 909) [order 2]
      (junction 901) -> (junction 910) : {VTQD_ACCSavedSetSpd_raw32 = KTQD_ACCActiveMetSpdHi_kph}
      (junction 902) -> (junction 911) [order 2]
      (junction 903) -> (junction 912) : {VTQD_ACCSavedSetSpd_raw32 = KTQD_ACCActiveMetSpdHiMPH_mph}
      (junction 910) -> (junction 909)
      (junction 912) -> (junction 911)
      (junction 909) -> (junction 913)
      (junction 911) -> (junction 914)
      (junction 913) -> (junction 914)
      (junction 914) -> (junction 915)
      (junction 906) -> (junction 907) [order 1] : [(VTQD_SWC2ScrollUpSta_enum == ENUM_SWCBOTTONPRESS_LONGPRESS ||...
          |   VTQD_SWC2ScrollDownSta_enum == ENUM_SWCBOTTONPRESS_LONGPRESS) &&...
          |  !VVMC_LVDAACCStatusInformation_flg && !VTQD_HoldResDet_flg]
          | %add20250114
      (junction 907) -> (junction 908) [order 1] : [VTQD_SWC2ScrollUpSta_enum == ENUM_SWCBOTTONPRESS_LONGPRESS]
      (junction 906) -> (junction 1200) [order 2]
      (junction 907) -> (junction 917) [order 2] : {VTQD_ACCSetSpd_raw32 = max(VTQD_ACCActiveMetSpdLo_raw32, ceil(VTQD_ACCSavedSetSpd_raw32 / VTQD_SetSpdDeltaLong_raw32 - ONE_FLOAT) * VTQD_SetSpdDeltaLong_raw32);
          |  VTQD_ACCSetSpd_raw32 = min (VTQD_ACCActiveMetSpdHi_raw32, VTQD_ACCSetSpd_raw32);
          |  VTQD_ACCSavedSetSpd_raw32 = VTQD_ACCSetSpd_raw32;
          |  VTQD_DistanceUnit_flg = VINP_Distanceunit_flg;}
      (junction 908) -> (junction 918) : {VTQD_ACCSetSpd_raw32 = min(VTQD_ACCActiveMetSpdHi_raw32, floor(VTQD_ACCSavedSetSpd_raw32 / VTQD_SetSpdDeltaLong_raw32 + ONE_FLOAT) * VTQD_SetSpdDeltaLong_raw32);
          |  VTQD_ACCSetSpd_raw32 = max (VTQD_ACCActiveMetSpdLo_raw32, VTQD_ACCSetSpd_raw32);
          |  VTQD_ACCSavedSetSpd_raw32 = VTQD_ACCSetSpd_raw32;
          |  VTQD_DistanceUnit_flg = VINP_Distanceunit_flg;}
      (junction 1200) -> (junction 1209) [order 1] : [(VTQD_SWC2ScrollUpSta_flg ||...
          |   VTQD_SWC2ScrollDownSta_flg) &&...
          |  VVMC_LVDAACCStatusInformation_flg]
          | %add20250114
      (junction 1200) -> (junction 1202) [order 2]
      (junction 1209) -> (junction 1207) : {VTQD_HoldResDet_flg = TRUE}
          | %add20250114
      (junction 1207) -> (junction 1202)
      (junction 1202) -> (junction 1204) : {VTQD_ACCSetSpd_raw32 = VTQD_ACCSavedSetSpd_raw32;
          |  VTQD_ACCSavedSetSpd_raw32 = VTQD_ACCSetSpd_raw32;
          |  VTQD_DistanceUnit_flg = VINP_Distanceunit_flg;}
      (junction 919) -> (junction 1278) [order 1] : [VINP_ADASACCSta_enum == ENUM_ADASACCSTA_OVERRIDE]
      (junction 1278) -> (junction 1266) [order 1] : [KTQD_ACCOVRDSpdAdj_flg &&...
          | (VTQD_Set2MeterSpd_flg ||...
          |  VTQD_SetRoadSpdLim_flg)]
      (junction 1266) -> (junction 1277) [order 1] : [VTQD_Set2MeterSpd_flg]
      (junction 919) -> (junction 924) [order 2] : {VTQD_ACCSetSpd_raw32 = VTQD_ACCSavedSetSpd_raw32;
          |  VTQD_ACCSavedSetSpd_raw32 = VTQD_ACCSetSpd_raw32;
          |  VTQD_DistanceUnit_flg = VINP_Distanceunit_flg;}
      (junction 1278) -> (junction 1268) [order 2]
      (junction 1266) -> (junction 1272) [order 2] : {VTQD_ACCSetSpd_raw32 =  min(VTQD_ACCActiveMetSpdHi_raw32, VTQD_SpdLim4SetSpd_raw32);
          |  VTQD_ACCSetSpd_raw32 = max(VTQD_ACCActiveMetSpdLo_raw32, VTQD_ACCSetSpd_raw32);
          |  VTQD_ACCSavedSetSpd_raw32 = VTQD_ACCSetSpd_raw32;
          |  VTQD_DistanceUnit_flg = VINP_Distanceunit_flg;}
      (junction 1277) -> (junction 1269) : {VTQD_ACCSetSpd_raw32 =  min(VTQD_ACCActiveMetSpdHi_raw32, VVMC_MeterIndSpeed_raw32);
          |  VTQD_ACCSetSpd_raw32 = max(VTQD_ACCActiveMetSpdLo_raw32, VTQD_ACCSetSpd_raw32);
          |  VTQD_ACCSavedSetSpd_raw32 = VTQD_ACCSetSpd_raw32;
          |  VTQD_DistanceUnit_flg = VINP_Distanceunit_flg;}
      (junction 1268) -> (junction 1280) [order 1] : [(VTQD_SWC2ScrollUpSta_enum == ENUM_SWCBOTTONPRESS_SHORTPRESS ||...
          |   VTQD_SWC2ScrollDownSta_enum == ENUM_SWCBOTTONPRESS_SHORTPRESS)]
      (junction 1280) -> (junction 1270) [order 1] : [VTQD_SWC2ScrollUpSta_enum == ENUM_SWCBOTTONPRESS_SHORTPRESS]
      (junction 1268) -> (junction 1276) [order 2]
      (junction 1280) -> (junction 1279) [order 2] : {VTQD_ACCSetSpd_raw32 =  min(VTQD_ACCActiveMetSpdHi_raw32, VTQD_ACCSavedSetSpd_raw32 - ONE_FLOAT);
          |  VTQD_ACCSetSpd_raw32 = max(VTQD_ACCActiveMetSpdLo_raw32, VTQD_ACCSetSpd_raw32);
          |  VTQD_ACCSavedSetSpd_raw32 = VTQD_ACCSetSpd_raw32;
          |  VTQD_DistanceUnit_flg = VINP_Distanceunit_flg;}
      (junction 1270) -> (junction 1274) : {VTQD_ACCSetSpd_raw32 =  min(VTQD_ACCActiveMetSpdHi_raw32, VTQD_ACCSavedSetSpd_raw32 + ONE_FLOAT);
          |  VTQD_ACCSetSpd_raw32 = max(VTQD_ACCActiveMetSpdLo_raw32, VTQD_ACCSetSpd_raw32);
          |  VTQD_ACCSavedSetSpd_raw32 = VTQD_ACCSetSpd_raw32;
          |  VTQD_DistanceUnit_flg = VINP_Distanceunit_flg;}
      (junction 1276) -> (junction 1285) [order 1] : [(VTQD_SWC2ScrollUpSta_enum == ENUM_SWCBOTTONPRESS_LONGPRESS ||...
          |   VTQD_SWC2ScrollDownSta_enum == ENUM_SWCBOTTONPRESS_LONGPRESS)]
      (junction 1285) -> (junction 1271) [order 1] : [VTQD_SWC2ScrollUpSta_enum == ENUM_SWCBOTTONPRESS_LONGPRESS]
      (junction 1276) -> (junction 1267) [order 2] : {VTQD_ACCSetSpd_raw32 = VTQD_ACCSavedSetSpd_raw32;
          |  VTQD_ACCSavedSetSpd_raw32 = VTQD_ACCSetSpd_raw32;
          |  VTQD_DistanceUnit_flg = VINP_Distanceunit_flg;}
      (junction 1285) -> (junction 1275) [order 2] : {VTQD_ACCSetSpd_raw32 = max(VTQD_ACCActiveMetSpdLo_raw32, ceil(VTQD_ACCSavedSetSpd_raw32 / VTQD_SetSpdDeltaLong_raw32 - ONE_FLOAT) * VTQD_SetSpdDeltaLong_raw32);
          |  VTQD_ACCSetSpd_raw32 = min (VTQD_ACCActiveMetSpdHi_raw32, VTQD_ACCSetSpd_raw32);
          |  VTQD_ACCSavedSetSpd_raw32 = VTQD_ACCSetSpd_raw32;
          |  VTQD_DistanceUnit_flg = VINP_Distanceunit_flg;}
      (junction 1271) -> (junction 1273) : {VTQD_ACCSetSpd_raw32 = min(VTQD_ACCActiveMetSpdHi_raw32, floor(VTQD_ACCSavedSetSpd_raw32 / VTQD_SetSpdDeltaLong_raw32 + ONE_FLOAT) * VTQD_SetSpdDeltaLong_raw32);
          |  VTQD_ACCSetSpd_raw32 = max (VTQD_ACCActiveMetSpdLo_raw32, VTQD_ACCSetSpd_raw32);
          |  VTQD_ACCSavedSetSpd_raw32 = VTQD_ACCSetSpd_raw32;
          |  VTQD_DistanceUnit_flg = VINP_Distanceunit_flg;}
    (default) -> RoadSpd.OFF_Error_Disable [order 3]
    RoadSpd.Terminal -> RoadSpd.OFF_Error_Disable [order 2] : [VINP_ADASACCSta_enum ~= ENUM_ADASACCSTA_ACTIVE &&...
        |  VINP_ADASACCSta_enum ~= ENUM_ADASACCSTA_OVERRIDE &&...
        |  VINP_ADASACCSta_enum ~= ENUM_ADASACCSTA_SHUTOFF]
    RoadSpd.OFF_Error_Disable -> RoadSpd.Terminal [order 2] : [VINP_ADASACCSta_enum == ENUM_ADASACCSTA_ACTIVE ||...
        |  VINP_ADASACCSta_enum == ENUM_ADASACCSTA_OVERRIDE ||...
        |  VINP_ADASACCSta_enum == ENUM_ADASACCSTA_SHUTOFF]
        | {VTQD_RoadSpdActive2Standby_flg = FALSE;}
    RoadSpd.Terminal -> RoadSpd.Active_Override_ShutOff [order 1] : [VINP_ADASACCSta_enum == ENUM_ADASACCSTA_ACTIVE ||...
        |  VINP_ADASACCSta_enum == ENUM_ADASACCSTA_OVERRIDE ||...
        |  VINP_ADASACCSta_enum == ENUM_ADASACCSTA_SHUTOFF]
    RoadSpd.Active_Override_ShutOff -> RoadSpd.Terminal [order 2] : [VINP_ADASACCSta_enum ~= ENUM_ADASACCSTA_ACTIVE &&...
        |  VINP_ADASACCSta_enum ~= ENUM_ADASACCSTA_OVERRIDE &&...
        |  VINP_ADASACCSta_enum ~= ENUM_ADASACCSTA_SHUTOFF]
    RoadSpd.OFF_Error_Disable -> RoadSpd.Standby [order 1] : [VINP_ADASACCSta_enum == ENUM_ADASACCSTA_STANDBY]
    RoadSpd.Standby -> RoadSpd.OFF_Error_Disable [order 2] : [VINP_ADASACCSta_enum ~= ENUM_ADASACCSTA_STANDBY]
        | {VTQD_RoadSpdActive2Standby_flg = FALSE;}
    RoadSpd.Active_Override_ShutOff -> RoadSpd.Standby [order 1] : [VINP_ADASACCSta_enum == ENUM_ADASACCSTA_STANDBY]
        | {VTQD_RoadSpdActive2Standby_flg = TRUE;}
    RoadSpd.Standby -> RoadSpd.Active_Override_ShutOff [order 1] : [VINP_ADASACCSta_enum == ENUM_ADASACCSTA_ACTIVE ||...
        |  VINP_ADASACCSta_enum == ENUM_ADASACCSTA_OVERRIDE ||...
        |  VINP_ADASACCSta_enum == ENUM_ADASACCSTA_SHUTOFF]
        | {VTQD_RoadSpdActive2Standby_flg = FALSE;}
    (default) -> RoadSpd.Active_Override_ShutOff [order 2] : [VINP_ADASACCSta_enum == ENUM_ADASACCSTA_ACTIVE ||...
        |  VINP_ADASACCSta_enum == ENUM_ADASACCSTA_OVERRIDE ||...
        |  VINP_ADASACCSta_enum == ENUM_ADASACCSTA_SHUTOFF]
    (default) -> RoadSpd.Standby [order 1] : [VINP_ADASACCSta_enum == ENUM_ADASACCSTA_STANDBY]
  (default) -> MeterSpd : {VTQD_ACCSavedSetSpd_raw32 = ZERO_FLOAT;
      |  VTQD_RoadSpdActive2Standby_flg = FALSE;
      |  VTQD_StandbyDisRoadSpd_flg = FALSE}
  RoadSpd -> MeterSpd : [!VINP_IVIACCAdaptiveSta_flg]
  MeterSpd -> RoadSpd : [VINP_IVIACCAdaptiveSta_flg]
  data: VINP_ADASACCSta_enum input; ENUM_ADASACCSTA_SHUTOFF parameter; ENUM_ADASACCSTA_STANDBY parameter; ENUM_ADASACCSTA_OVERRIDE parameter; ENUM_ADASACCSTA_ACTIVE parameter; ZERO_FLOAT parameter; VTQD_ACCSetSpd_raw32 output single; VINP_IVIACCAdaptiveSta_flg input; VTQD_SpdLim4SetSpd_raw32 input; VTQD_ACCActiveMetSpdHi_raw32 input; VTQD_ACCActiveMetSpdLo_raw32 input; VTQD_Set2MeterSpd_flg input; VTQD_SWC2ScrollUpSta_enum input; VTQD_SWC2ScrollDownSta_enum input; ENUM_SWCBOTTONPRESS_SHORTPRESS parameter; ONE_FLOAT parameter; ENUM_SWCBOTTONPRESS_LONGPRESS parameter; VTQD_ACCSavedSetSpd_raw32 local single; VTQD_SetSpdDeltaLong_raw32 input; VTQD_SetRoadSpdLim_flg input; KTQD_ACCOVRDSpdAdj_flg parameter; KPH2MPH parameter; VTQD_DistanceUnit_flg local boolean; MPH2KPH parameter; KTQD_ACCActiveMetSpdHiMPH_mph parameter; KTQD_ACCActiveMetSpdHi_kph parameter; KTQD_ACCActiveMetSpdLoMPH_mph parameter; KTQD_ACCActiveMetSpdLo_kph parameter; VTQD_RoadSpdActive2Standby_flg local boolean; VINP_Distanceunit_flg input; VTQD_ADASSLIFSpdLimDet_flg input; VTQD_StandbyDisRoadSpd_flg local boolean; VTQD_LScrollPressShort_flg input; FALSE parameter; TRUE parameter; ENUM_SWCBOTTONPRESS_NOPRESS parameter; VVMC_LVDAACCStatusInformation_flg input; VVMC_MeterIndSpeed_raw32 input; VTQD_SWC2ScrollUpSta_flg input; VTQD_SWC2ScrollDownSta_flg input; VTQD_HoldResDet_flg local boolean; VTQD_LastSetSpd_kph input
